simulink model "Three_Phase_RLE"  (R2021b)
settings: Solver=VariableStepAuto  StartTime=0.0  StopTime=1  MaxStep=1e-4  RelTol=1e-3
InitFcn:
  | v=300
  | a=0
  | b=60
  | c=120
  | d=180
  | e=240
  | g=300
  | 
  | f=50
  | p=50
  | pe=0.02
  | t=5
libraries: spsThyristorLib x6, spsThreePhaseVIMeasurementLib x1, spsDCVoltageSourceLib x1, spsDCMachineLib x1, spsGroundLib x1, spsThreePhaseProgrammableVoltageSourceLib x1, spsVoltageMeasurementLib x1, spspowerguiLib x1
settings Model: Creator=dell  LastModifiedBy=viraj
settings SolverCC: AlgebraicLoopSolver=TrustRegion
settings DataIOCC: ReturnWorkspaceOutputs=off
settings DebuggingCC: SFMachineParentedDataDiag=warning  ArithmeticOperatorsInVariantConditions=warning
settings SFSimCC: SimUseLocalCustomCode=off  CustomCodeUndefinedFunction=UseInterfaceOnly
settings RTWCC: RTWUseLocalCustomCode=off
settings CodeAppCC: StateflowObjectComments=on
settings SimscapeCC: SimscapeNormalizeSystem=off

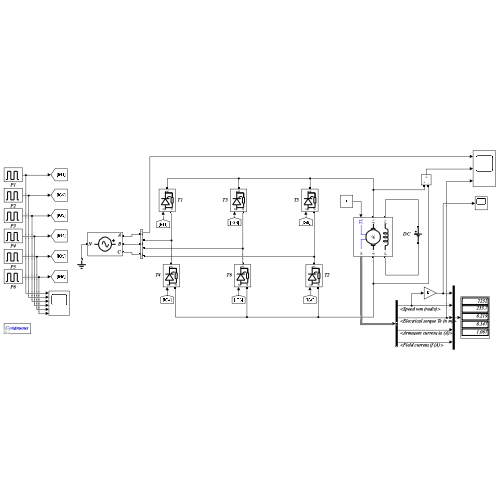
[thumbnail: Simulink's stored preview of the top-level diagram]
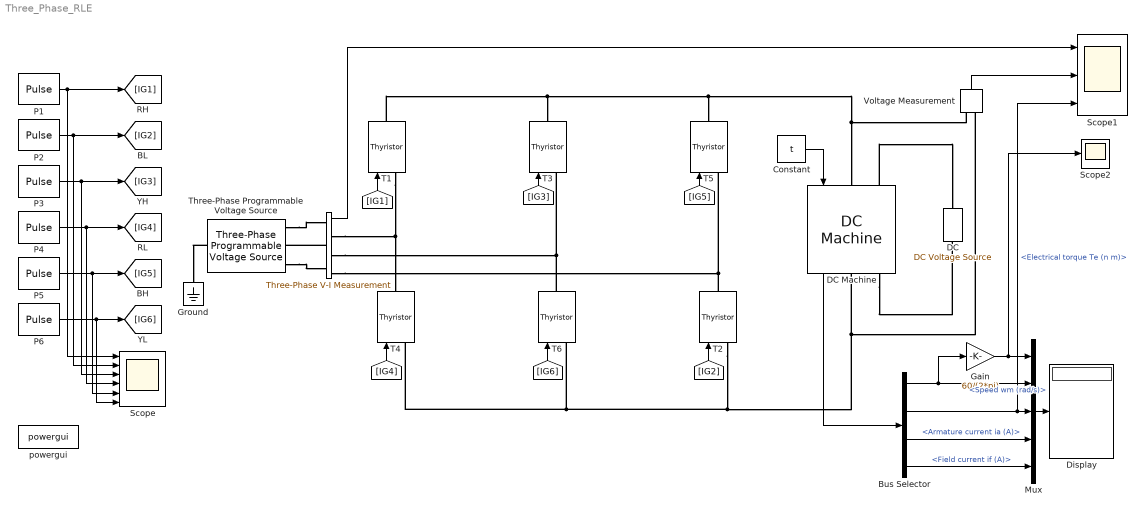
== system Three_Phase_RLE ==
  "         " : spsThreePhaseVIMeasurementLib/Three-Phase V-I Measurement  VoltageMeasurement=phase-to-ground  SetLabelV=off  LabelV=Vabc  Vpu=off  VpuLL=off  CurrentMeasurement=no  SetLabelI=off  LabelI=Iabc  Ipu=off  Pbase=100e6  Vbase=500e3  OutputType=Complex  PhasorSimulation=off  PSBequivalent=0
  Bus Selector : BusSelector  OutputSignals=Speed wm (rad/s),Electrical torque Te (n m),Armature current ia (A),Field current if (A)
  Constant : Constant  Value=t
  "DC " : spsDCVoltageSourceLib/DC Voltage Source  Amplitude=v  Measurements=None
  DC Machine : spsDCMachineLib/DC Machine  PresetModel=01: 5HP 240V 1750RPM Field:300V  MechanicalLoad=Torque TL  FieldType=Wound  ShowDetailedParameters=on  MeasurementBus=off  RLa=[2.581 0.028]  RLf=[281.2 156]  Laf=0.9483  MachineConstant=Torque constant (N.m/A)  Ke=1.8  Kt=1.8  J=0.02215  Bm=0.002953  Tf=0.5161  w0=0  Ifinit=1.06685632871799  TsPowergui=0  TsBlock=-1
  Display : Display
  Gain : Gain  Gain=60/(2*pi)
  Ground : spsGroundLib/Ground  LConnTagsString=a
  Mux : Mux  Inputs=5
  P1 : DiscretePulseGenerator  PulseType=Time based  Period=1/f  PulseWidth=p  PhaseDelay=((pe*a)/360)
  P2 : DiscretePulseGenerator  PulseType=Time based  Period=1/f  PulseWidth=p  PhaseDelay=((pe*b)/360)
  P3 : DiscretePulseGenerator  PulseType=Time based  Period=1/f  PulseWidth=p  PhaseDelay=((pe*c)/360)
  P4 : DiscretePulseGenerator  PulseType=Time based  Period=1/f  PulseWidth=p  PhaseDelay=((pe*d)/360)
  P5 : DiscretePulseGenerator  PulseType=Time based  Period=1/f  PulseWidth=p  PhaseDelay=((pe*e)/360)
  P6 : DiscretePulseGenerator  PulseType=Time based  Period=1/f  PulseWidth=p  PhaseDelay=((pe*g)/360)
  Scope : Scope  NumInputPorts=6
  Scope1 : Scope  NumInputPorts=3
  Scope2 : Scope
  T{1..6} (6 alike) : spsThyristorLib/Thyristor  Ron=0.001  Lon=0  Vf=0.8  IC=0  Rs=500  Cs=250e-9  Measurements=off
  Three-Phase Programmable Voltage Source : spsThreePhaseProgrammableVoltageSourceLib/Three-Phase Programmable Voltage Source  PositiveSequence=[188 0 50]  VariationEntity=None  VariationType=Step  VariationTypeAlt=Step  VariationStep=0.5  VariationRate=10  VariationMagnitude=0.3  VariationFrequency=2  VariationTiming=[1 2]  VariationPhaseA=off  Amplitudes=[1 0.8 1.2 1.0]  TimeValues=[0 0.1 0.15 0.2]  HarmonicGeneration=off  HarmonicA=[3 0.2 -25 0]  HarmonicB=[2 0.15 35 2]  Timing="[0.05  3]"  BusType=swing  Pref=0  Qref=0  Qmin=-inf  Qmax=inf
  Voltage Measurement : spsVoltageMeasurementLib/Voltage Measurement  PhasorSimulation=off  OutputType=Complex  PSBequivalent=0
  powergui : spspowerguiLib/powergui  Priority=1  SimulationMode=Continuous  SampleTime=50e-6  frequency=60  Iterations=50  frequencyindice=0  Pbase=100e6  ErrMax=1e-4  UnitsV=kV  UnitsW=MW  buscounter=0  FunctionMessages=off  echomessages=off  EnableUseOfTLC=off  CurrentSourceSwitches=off  DisableSnubberDevices=off  DisableRonSwitches=off  DisableVfSwitches=off  DisplayEquations=off  AutomaticDiscreteSolvers=off  SolverType=Tustin/Backward Euler (TBE)  Interpol=off  ExternalGateDelay=off  methode=off  Ts=100  x0status=blocks  SPID=on  SwTol=0  HookPort=off  NonlinearTolerance=1e-4  nMaxIteration=100  ContinueOnMaxIteration=off  RestoreLinks=warning  ResistiveCurrentMeasurement=off  Frange=[0:2:500]  Ylog=off  Xlog=on  ShowGrid=off  save=off  variable=ZData  structure=GG  ZoomFFT=off  StartTime=0.02  cycles=1  DisplayStyle=1  fundamental=25  FreqAxis=on  MaxFrequency=1000  frequencyindicesteady=1  RmsSteady=1  display=off
  wires:
  DC Machine/1 -> Bus Selector/1
  "         "/1 -> Scope1/1
  P4/1 -> [IG4], Scope/4
  Constant/1 -> DC Machine/1
  [IG4] -> T4/1
  P1/1 -> [IG1], Scope/1
  Bus Selector/4 -> Mux/5  "<Field current if (A)>"
  Bus Selector/2 -> Scope1/3, Mux/3  "<Electrical torque Te (n m)>"
  [IG6] -> T6/1
  Bus Selector/1 -> Gain/1, Mux/2  "<Speed wm (rad/s)>"
  [IG2] -> T2/1
  Bus Selector/3 -> Mux/4  "<Armature current ia (A)>"
  Mux/1 -> Display/1
  P2/1 -> [IG2], Scope/2
  Voltage Measurement/1 -> Scope1/2
  P6/1 -> [IG6], Scope/6
  [IG1] -> T1/1
  P5/1 -> [IG5], Scope/5
  Gain/1 -> Scope2/1, Mux/1
  [IG5] -> T5/1
  P3/1 -> [IG3], Scope/3
  [IG3] -> T3/1
  connections:
  T6/LConn1 -- T4/LConn1 -- Voltage Measurement/LConn2 -- DC Machine/RConn1 -- T2/LConn1
  T6/RConn1 -- "         "/RConn2 -- T3/LConn1
  T2/RConn1 -- "         "/RConn3 -- T5/LConn1
  T1/RConn1 -- T3/RConn1 -- DC Machine/LConn1 -- Voltage Measurement/LConn1 -- T5/RConn1
  T1/LConn1 -- T4/RConn1 -- "         "/RConn1
  Three-Phase Programmable Voltage Source/LConn1 -- Ground/LConn1
  DC Machine/LConn2 -- "DC "/RConn1
  DC Machine/RConn2 -- "DC "/LConn1
  "         "/LConn2 -- Three-Phase Programmable Voltage Source/RConn2
  Three-Phase Programmable Voltage Source/RConn1 -- "         "/LConn1
  Three-Phase Programmable Voltage Source/RConn3 -- "         "/LConn3
